simulink model "LgrstOpnFlow"  (R2018b)
settings: Solver=FixedStepDiscrete  StartTime=0.0  StopTime=10.0  FixedStep=0.01  RelTol=1e-3
settings Model: ModifiedHistory=2025.11.03 V2.0.1 腿托只发送目标位置，不做逻辑  Creator=sn2xws  LastModifiedBy=sn55gm
settings DataIOCC: SaveFormat=StructureWithTime
settings OptimizationCC: DefaultParameterBehavior=Inlined  EnhancedBackFolding=on  PassReuseOutputArgsAs=Individual arguments  ZeroExternalMemoryAtStartup=off  ZeroInternalMemoryAtStartup=off  OptimizeBlockOrder=speed  DifferentSizesBufferReuse=on  OptimizationCustomize=off
settings DebuggingCC: ParameterTunabilityLossMsg=error
settings SFSimCC: MATLABDynamicMemAlloc=off
settings RTWCC: SystemTargetFile=autosar.tlc  GenCodeOnly=on  TemplateMakefile=ert_default_tmf  Description=AUTOSAR  GenerateReport=on  IncludeHyperlinkInReport=on  LaunchReport=on  GenerateTraceInfo=on  GenerateTraceReport=on  GenerateTraceReportSl=on  GenerateTraceReportSf=on  GenerateTraceReportEml=on  GenerateCodeMetricsReport=on
settings CodeAppCC: ForceParamTrailComments=on  IgnoreCustomStorageClasses=off  OperatorAnnotations=on  SimulinkDataObjDesc=on  SFDataObjDesc=on  InsertBlockDesc=on
settings STFCustomTargetCC: TargetLangStandard=C99 (ISO)  MultiwordLength=256  ParMdlRefBuildCompliant=on  CompOptLevelCompliant=on  IncludeMdlTerminateFcn=off  CombineOutputUpdateFcns=on  SuppressErrorStatus=on  ERTCustomFileBanners=on  SupportNonFinite=off  SupportComplex=off  SupportContinuousTime=off  SupportNonInlinedSFcns=off  RemoveResetFunc=on  MATLABClassNameForMDSCustomization=Simulink.SoftwareTarget.ERTCustomization  AutosarCompliant=on  UseToolchainInfoCompliant=on  LookupTableObjectStructAxisOrder=2,1,3,4,...  LUTObjectStructOrderEvenSpacing=Size,Table,Breakpoints  SystemTargetFile=autosar.tlc
settings ERTTargetCC: TargetLangStandard=C99 (ISO)  ConcurrentExecutionCompliant=off  IncludeMdlTerminateFcn=off  SuppressErrorStatus=on  SupportNonFinite=off  SupportComplex=off  ModelStepFunctionPrototypeControlCompliant=off  CPPClassGenCompliant=off  AutosarCompliant=on  LookupTableObjectStructAxisOrder=2,1,3,4,...  LUTObjectStructOrderEvenSpacing=Size,Table,Breakpoints  InlinedParameterPlacement=NonHierarchical  ERTCustomFileTemplate=example_file_process.tlc  ERTFilePackagingFormat=Compact

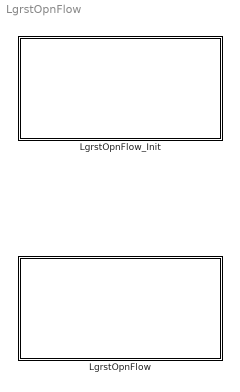
== system LgrstOpnFlow ==
  LgrstOpnFlow : Subsystem
  LgrstOpnFlow_Init : Subsystem

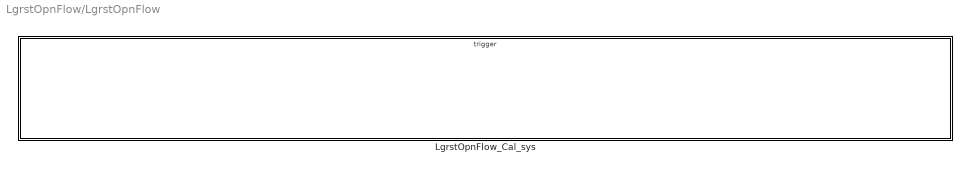
== system LgrstOpnFlow/LgrstOpnFlow ==
  LgrstOpnFlow_Cal_sys : Subsystem

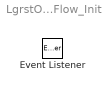
== system LgrstOpnFlow/LgrstOpnFlow_Init ==
  Event Listener : EventListener  EventName=reset

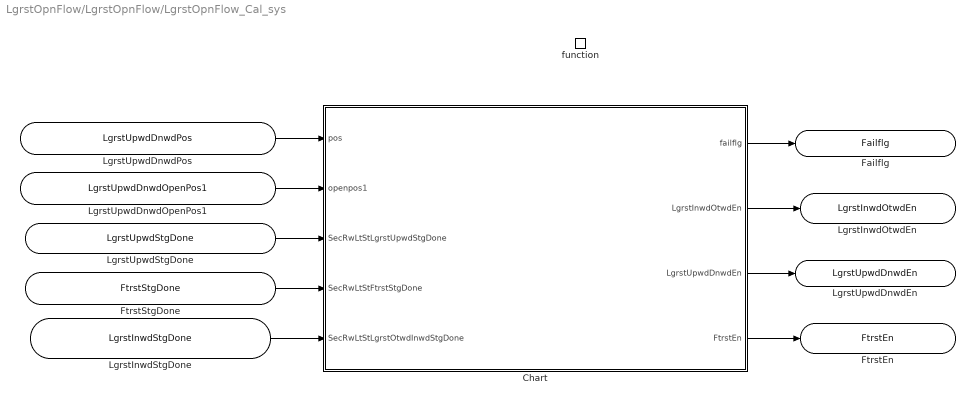
== system LgrstOpnFlow/LgrstOpnFlow/LgrstOpnFlow_Cal_sys ==
  function : TriggerPort  TriggerType=function-call  IsSimulinkFunction=on  FunctionName=LgrstOpnFlow_Cal  VariantControl=(inherit)
  Chart : Stateflow chart  TreatAsAtomicUnit=on
  LgrstUpwdDnwdPos : ArgIn  OutDataTypeStr=uint16  ArgumentName=LgrstUpwdDnwdPos
  LgrstUpwdDnwdOpenPos1 : ArgIn  Port=2  OutDataTypeStr=uint16  ArgumentName=LgrstUpwdDnwdOpenPos1
  LgrstUpwdStgDone : ArgIn  Port=3  OutDataTypeStr=boolean  ArgumentName=LgrstUpwdStgDone
  FtrstStgDone : ArgIn  Port=4  OutDataTypeStr=boolean  ArgumentName=FtrstStgDone
  LgrstInwdStgDone : ArgIn  Port=5  OutDataTypeStr=boolean  ArgumentName=LgrstInwdStgDone
  Failflg : ArgOut  OutDataTypeStr=boolean  ArgumentName=Failflg
  LgrstInwdOtwdEn : ArgOut  Port=2  OutDataTypeStr=boolean  ArgumentName=LgrstInwdOtwdEn
  LgrstUpwdDnwdEn : ArgOut  Port=3  OutDataTypeStr=boolean  ArgumentName=LgrstUpwdDnwdEn
  FtrstEn : ArgOut  Port=4  OutDataTypeStr=boolean  ArgumentName=FtrstEn
  wires:
  LgrstUpwdDnwdPos/1 -> Chart/1(pos)
  LgrstUpwdDnwdOpenPos1/1 -> Chart/2(openpos1)
  LgrstUpwdStgDone/1 -> Chart/3(SecRwLtStLgrstUpwdStgDone)
  FtrstStgDone/1 -> Chart/4(SecRwLtStFtrstStgDone)
  LgrstInwdStgDone/1 -> Chart/5(SecRwLtStLgrstOtwdInwdStgDone)
  Chart/4(FtrstEn) -> FtrstEn/1
  Chart/3(LgrstUpwdDnwdEn) -> LgrstUpwdDnwdEn/1
  Chart/2(LgrstInwdOtwdEn) -> LgrstInwdOtwdEn/1
  Chart/1(failflg) -> Failflg/1

== stateflow chart LgrstOpnFlow/LgrstOpnFlow_Cal_sys/Chart ==
  (default) -> (junction 64) : {
      | failflg =0;
      | LgrstInwdOtwdEn=0;
      | LgrstUpwdDnwdEn=0;
      | FtrstEn = 0;
      | }
  (junction 64) -> (junction 74) [order 1] : [SecRwLtStLgrstUpwdStgDone]
  (junction 64) -> (junction 66) [order 2] : {
      | LgrstUpwdDnwdEn=1;
      | }
  (junction 74) -> (junction 102)
  (junction 102) -> (junction 66)
  (junction 66) -> (junction 113)
  (junction 113) -> (junction 115) [order 1] : [SecRwLtStLgrstOtwdInwdStgDone]
  (junction 113) -> (junction 116) [order 2] : {
      | LgrstInwdOtwdEn=1;
      | }
  (junction 115) -> (junction 122)
  (junction 122) -> (junction 116)
  (junction 116) -> (junction 166)
  data: pos input uint16; openpos1 input uint16; SecRwLtStLgrstUpwdStgDone input boolean; SecRwLtStFtrstStgDone input boolean; SecRwLtStLgrstOtwdInwdStgDone input boolean; failflg output boolean; LgrstInwdOtwdEn output boolean; LgrstUpwdDnwdEn output boolean; FtrstEn output boolean
